simulink model "Entrega_1"  (R2022a)
settings: Solver=VariableStepAuto  StartTime=0.0  StopTime=5  RelTol=1e-3
libraries: simulink x2
settings Model: Creator=diego  LastModifiedBy=diego

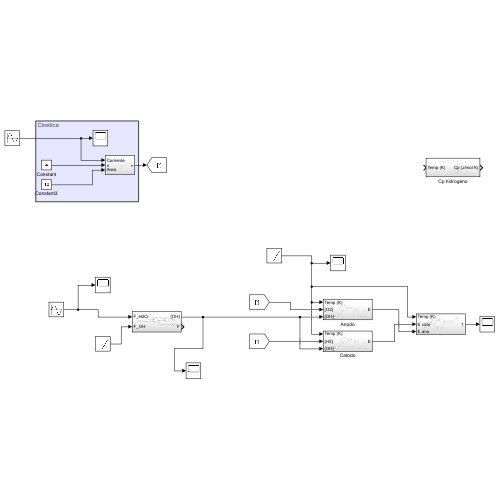
[thumbnail: Simulink's stored preview of the top-level diagram]
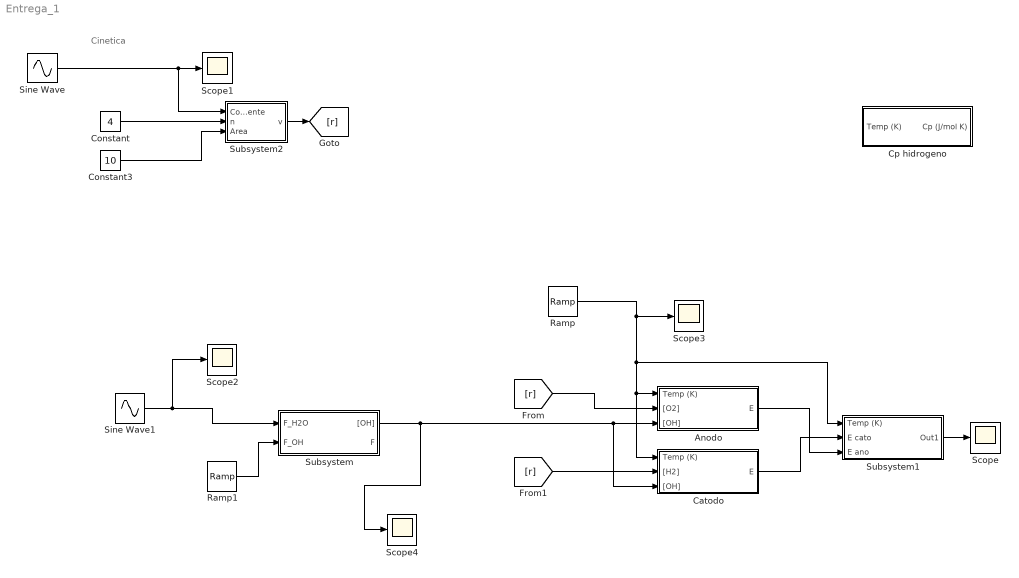
== system Entrega_1 ==
  note: Cinetica
  Anodo : Subsystem
  Catodo : Subsystem
  Constant : Constant  Value=4  VectorParams1D=off  SampleTime=-1
  Constant3 : Constant  Value=10  VectorParams1D=off  SampleTime=-1
  Cp hidrogeno : Subsystem
  Ramp : simulink/Sources/Ramp  slope=10  start=0  InitialOutput=273.15
  Ramp1 : simulink/Sources/Ramp  slope=200  start=0  InitialOutput=0
  Scope{,1..4} (5 alike) : Scope
  Sine Wave : Sin  Amplitude=0.01  Bias=3  Frequency=2  SampleTime=0
  Sine Wave1 : Sin  Amplitude=8  Bias=100  Frequency=5  SampleTime=0
  Subsystem : Subsystem
  Subsystem1 : Subsystem
  Subsystem2 : Subsystem
  wires:
  Anodo/1(E) -> Subsystem1/3(E ano)
  [r] -> Anodo/2("[O2]")
  [r] -> Catodo/2("[H2]")
  Subsystem/1("[OH]") -> Scope4/1, Catodo/3("[OH]"), Anodo/3("[OH]")
  Catodo/1(E) -> Subsystem1/2(E cato)
  Sine Wave1/1 -> Scope2/1, Subsystem/1(F_H2O)
  Ramp1/1 -> Subsystem/2(F_OH)
  Subsystem1/1(Out1) -> Scope/1
  Constant/1 -> Subsystem2/2(n)
  Constant3/1 -> Subsystem2/3(Area)
  Sine Wave/1 -> Subsystem2/1(Corriente), Scope1/1
  Subsystem2/1(v) -> [r]
  Ramp/1 -> Scope3/1, Subsystem1/1(Temp (K)), Anodo/1(Temp (K)), Catodo/1(Temp (K))

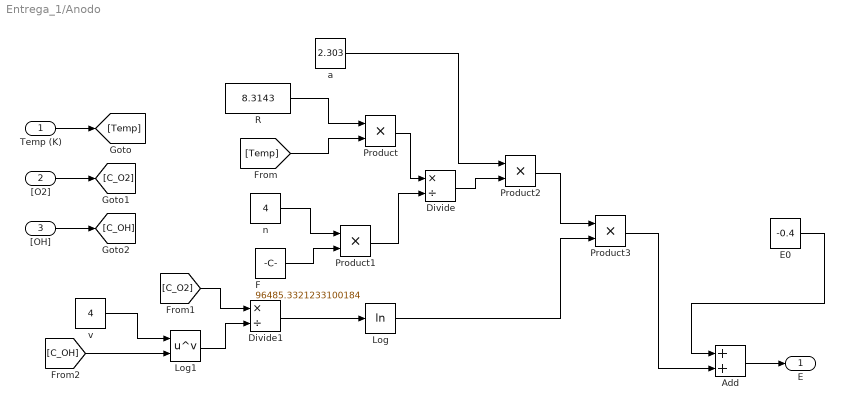
== system Entrega_1/Anodo ==
  Temp (K) : Inport
  "[O2]" : Inport  Port=2
  "[OH]" : Inport  Port=3
  Add : Sum
  Divide : Product  Inputs=*/
  Divide1 : Product  Inputs=*/
  E0 : Constant  Value=-0.4
  F : Constant  Value=96485.3321233100184
  Log : Math  Operator=log
  Log1 : Math  Operator=pow
  Product{,1..3} (4 alike) : Product
  R : Constant  Value=8.3143
  a : Constant  Value=2.303
  n : Constant  Value=4
  v : Constant  Value=4
  E : Outport
  wires:
  Temp (K)/1 -> [Temp]
  "[O2]"/1 -> [C_O2]
  "[OH]"/1 -> [C_OH]
  E0/1 -> Add/1
  [Temp] -> Product/2
  R/1 -> Product/1
  n/1 -> Product1/1
  F/1 -> Product1/2
  Product1/1 -> Divide/2
  Product/1 -> Divide/1
  Divide/1 -> Product2/2
  a/1 -> Product2/1
  [C_OH] -> Log1/2
  v/1 -> Log1/1
  [C_O2] -> Divide1/1
  Log1/1 -> Divide1/2
  Divide1/1 -> Log/1
  Log/1 -> Product3/2
  Product2/1 -> Product3/1
  Product3/1 -> Add/2
  Add/1 -> E/1

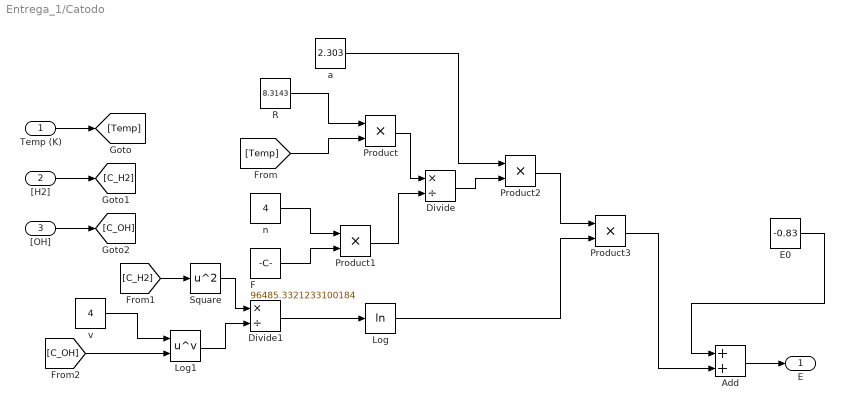
== system Entrega_1/Catodo ==
  Temp (K) : Inport
  "[H2]" : Inport  Port=2
  "[OH]" : Inport  Port=3
  Add : Sum
  Divide : Product  Inputs=*/
  Divide1 : Product  Inputs=*/
  E0 : Constant  Value=-0.83
  F : Constant  Value=96485.3321233100184
  Log : Math  Operator=log
  Log1 : Math  Operator=pow
  Product{,1..3} (4 alike) : Product
  R : Constant  Value=8.3143
  Square : Math  Operator=square
  a : Constant  Value=2.303
  n : Constant  Value=4
  v : Constant  Value=4
  E : Outport
  wires:
  Add/1 -> E/1
  Product3/1 -> Add/2
  Product2/1 -> Product3/1
  Log/1 -> Product3/2
  Divide1/1 -> Log/1
  Log1/1 -> Divide1/2
  [C_H2] -> Square/1
  v/1 -> Log1/1
  [C_OH] -> Log1/2
  a/1 -> Product2/1
  Divide/1 -> Product2/2
  Product/1 -> Divide/1
  Product1/1 -> Divide/2
  F/1 -> Product1/2
  n/1 -> Product1/1
  R/1 -> Product/1
  [Temp] -> Product/2
  E0/1 -> Add/1
  "[OH]"/1 -> [C_OH]
  "[H2]"/1 -> [C_H2]
  Temp (K)/1 -> [Temp]
  Square/1 -> Divide1/1

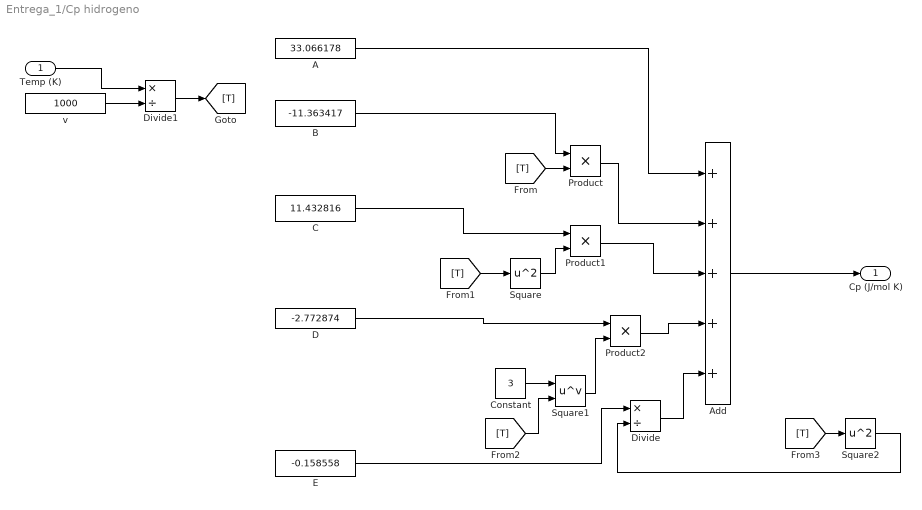
== system Entrega_1/Cp hidrogeno ==
  Temp (K) : Inport
  A : Constant  Value=33.066178
  Add : Sum  Inputs=+++++
  B : Constant  Value=-11.363417
  C : Constant  Value=11.432816
  Constant : Constant  Value=3
  D : Constant  Value=-2.772874
  Divide : Product  Inputs=*/
  Divide1 : Product  Inputs=*/
  E : Constant  Value=-0.158558
  Product : Product
  Product1 : Product
  Product2 : Product
  Square : Math  Operator=square
  Square1 : Math  Operator=pow
  Square2 : Math  Operator=square
  v : Constant  Value=1000
  Cp (J/mol K) : Outport
  wires:
  Temp (K)/1 -> Divide1/1
  B/1 -> Product/1
  [T] -> Product/2
  [T] -> Square/1
  C/1 -> Product1/1
  Square/1 -> Product1/2
  [T] -> Square1/2
  Constant/1 -> Square1/1
  Square2/1 -> Divide/2
  [T] -> Square2/1
  E/1 -> Divide/1
  A/1 -> Add/1
  Product/1 -> Add/2
  Product1/1 -> Add/3
  D/1 -> Product2/1
  Square1/1 -> Product2/2
  Product2/1 -> Add/4
  Divide/1 -> Add/5
  Add/1 -> Cp (J/mol K)/1
  v/1 -> Divide1/2
  Divide1/1 -> [T]

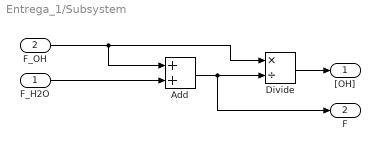
== system Entrega_1/Subsystem ==
  F_H2O : Inport
  F_OH : Inport  Port=2
  Add : Sum
  Divide : Product  Inputs=*/
  "[OH]" : Outport
  F : Outport  Port=2
  wires:
  F_H2O/1 -> Add/2
  F_OH/1 -> Divide/1, Add/1
  Add/1 -> F/1, Divide/2
  Divide/1 -> "[OH]"/1

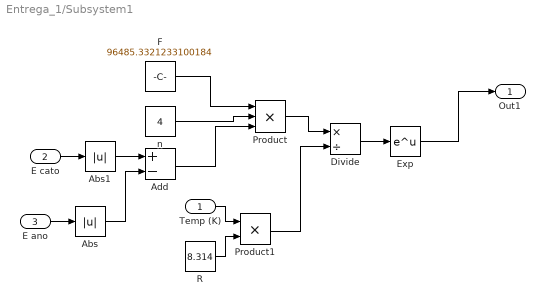
== system Entrega_1/Subsystem1 ==
  Temp (K) : Inport
  E cato : Inport  Port=2
  E ano : Inport  Port=3
  Abs : Abs  SaturateOnIntegerOverflow=off
  Abs1 : Abs  SaturateOnIntegerOverflow=off
  Add : Sum  Inputs=+-
  Divide : Product  Inputs=*/
  Exp : Math
  F : Constant  Value=96485.3321233100184
  Product : Product  Inputs=3
  Product1 : Product
  R : Constant  Value=8.314
  n : Constant  Value=4
  Out1 : Outport
  wires:
  F/1 -> Product/1
  n/1 -> Product/2
  Add/1 -> Product/3
  Product/1 -> Divide/1
  Temp (K)/1 -> Product1/1
  R/1 -> Product1/2
  Product1/1 -> Divide/2
  Divide/1 -> Exp/1
  Exp/1 -> Out1/1
  E ano/1 -> Abs/1
  Abs/1 -> Add/2
  Abs1/1 -> Add/1
  E cato/1 -> Abs1/1

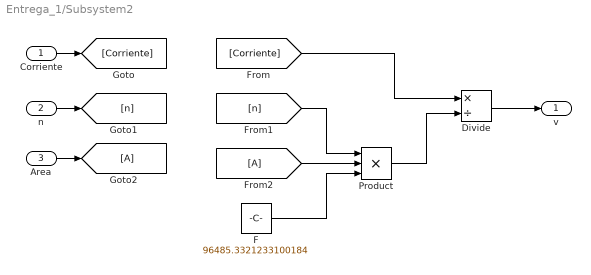
== system Entrega_1/Subsystem2 ==
  Corriente : Inport
  n : Inport  Port=2
  Area : Inport  Port=3
  Divide : Product  Inputs=*/
  F : Constant  Value=96485.3321233100184
  From2 : From
  Goto2 : Goto
  Product : Product  Inputs=3
  v : Outport
  wires:
  Corriente/1 -> [Corriente]
  n/1 -> [n]
  Area/1 -> Goto2/1
  [n] -> Product/1
  From2/1 -> Product/2
  F/1 -> Product/3
  [Corriente] -> Divide/1
  Product/1 -> Divide/2
  Divide/1 -> v/1
